simulink model "hysteresis_phenomenon"  (R2021a)
settings: Solver=ode5  StartTime=0.0  StopTime=10.0  FixedStep=0.001  RelTol=1e-3
settings Model: Creator=a1752760  LastModifiedBy=a1752760
settings SolverCC: AlgebraicLoopSolver=TrustRegion
settings DataIOCC: ReturnWorkspaceOutputs=off
settings DebuggingCC: SFMachineParentedDataDiag=warning  ArithmeticOperatorsInVariantConditions=warning
settings SFSimCC: CustomCodeUndefinedFunction=UseInterfaceOnly

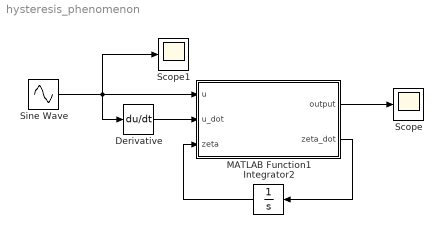
== system hysteresis_phenomenon ==
  Derivative : Derivative
  Integrator2 : Integrator  ContinuousStateAttributes='speed'
  MATLAB Function1 : MATLAB Function  TreatAsAtomicUnit=on
  Scope : Scope
  Scope1 : Scope
  Sine Wave : Sin  Amplitude=3  Frequency=2  SampleTime=0
  wires:
  MATLAB Function1/2(zeta_dot) -> Integrator2/1
  Integrator2/1 -> MATLAB Function1/3(zeta)
  Sine Wave/1 -> Scope1/1, Derivative/1, MATLAB Function1/1(u)
  Derivative/1 -> MATLAB Function1/2(u_dot)
  MATLAB Function1/1(output) -> Scope/1

== matlab function hysteresis_phenomenon/MATLAB Function1 ==
  data: u input; output output; u_dot input; zeta input; zeta_dot output
function [output,zeta_dot] = B_W_hysteresis(u, u_dot, zeta)

mu=1.5;
mu_bar=3;
chi_bar=1;
chi=0.5;
n=2;

output=mu*u+mu_bar*zeta;

f=1-chi_bar*sign(u_dot).*abs(zeta).^(n-1).*zeta-chi*abs(zeta).^n;

zeta_dot=u_dot.*f;

end
